simulink model "StateMachine_v3"  (R2015a)
settings: Solver=ode1  StartTime=0.0  StopTime=Inf  FixedStep=0.001  RelTol=1e-3
PostLoadFcn:
  | , if any(exist('dsrtsu_mdlpostloadfcn', 'file') == [2, 3, 6]), try dsrtsu_mdlpostloadfcn('Execute', bdroot); catch fprintf('Error in PostLoadFcn (dsrtsu_mdlpostloadfcn) for model "%s":\n %s\n', bdroot, lasterr); end, end,
libraries: rtican x25, rti1401lib_adc_type4 x16, rti1401lib_dio_type3 x16, rtilib1401 x1
(part 4 of 6)

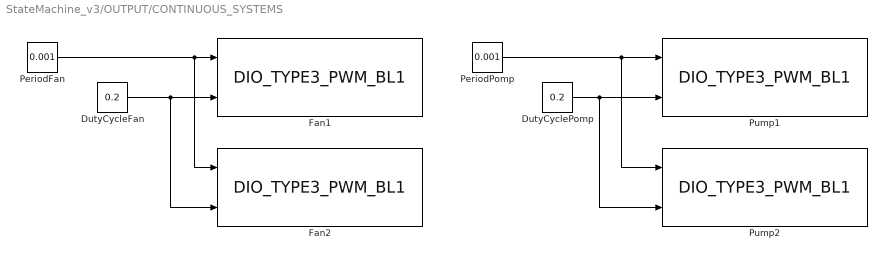
== system StateMachine_v3/OUTPUT/CONTINUOUS_SYSTEMS ==
  DutyCycleFan : Constant  Value=0.2
  DutyCyclePomp : Constant  Value=0.2
  Fan1 : rti1401lib_dio_type3/DIO_TYPE3_PWM_BL1  DSProperties=struct('RTI',struct('Version',uint32(2),'BlockType',struct('isSLSource',uint8(0),'isSLSink',uint8(1),'isHWSource',uint8(0),'isHWSink',uint8(1),'isSetup',uint8(0),'isInline',uint8(1),'isNonInline',uint8(0),'isInterrupt',uint8(0),'isChannelwise',uint8(1)),'IOBoardType',{{'DS1401','STD','DIOT3'}},'UnitType','PWM','Identifier','PWM','DialogType','ML','BlockSet','NONE','SlaveProcessor','NONE'))  RTIBlockInterface=struct('InputPortsWidth',int32([1 1]),'InputPortsActive',[1 1],'InputPortsName',{{'Period',['Duty Cycle']}},'BlockDisplay',{{['DIO TP3 PWM\nModule: 1\nPort: 1\nChannel: 3'],'center'}},'IconTransparency','on','InitLevel',3,'DialogFcn','rti1401stddiot3pwmgui','BlockName',struct('Token',{{'DIO_TYPE3_PWM_BL1'}}))  RTIBlockParameters=struct('ModuleNo',{{1,'OFF',[1 16]}},'PortNo',{{1,'OFF',[1 3]}},'ChannelNo',{{3,'OFF',[1 16]}},'SupplyRailsCh',{{[1 1],'OFF',[0 1 0 1]}},'UpdateMode',{{1,'ON',[1 2]}},'PeriodRange',{{7,'OFF',[1 16]}},'DutyCycleInit',{{'0','OFF',[0 1]}},'PeriodInit',{{'5e-05','OFF',[]}},'TerminationMode',{{0,'OFF',[0 1]}},'OutputTermValidate',{{0,'OFF',[0 1]}},'OutputTermBuildCheck',{{0,'OFF',[]}},'DutyCycleTerm',{{'0','OFF',[0 1]}},'PeriodTerm',{{'5e-05','OFF',[]}},'TLCFileName',{{'rti1401dio_t3_pwm','OFF',[]}},'EnableInterrupt',{{0,'OFF',[0 1]}},'TriggerEdgeType',{{1,'OFF',[1 3]}})  RTISFcnParameters=struct('ModuleNo','int32','PortNo','int16','ChannelNo','int16','SupplyRailsCh','int16','UpdateMode','int16','PeriodRange','int16','DutyCycleInit','double','PeriodInit','double','TerminationMode','int16','OutputTermValidate','int16','DutyCycleTerm','double','PeriodTerm','double','TLCFileName','char','EnableInterrupt','int16','TriggerEdgeType','int32')  RTIBlockParaDefault=struct('ModuleNo',1,'PortNo',1,'ChannelNo',1,'SupplyRailsCh',[1 1],'UpdateMode',1,'PeriodRange',7,'DutyCycleInit',0,'PeriodInit',5e-05,'TerminationMode',0,'OutputTermValidate',0,'OutputTermBuildCheck',0,'DutyCycleTerm',0,'PeriodTerm',5e-05,'TLCFileName','rti1401dio_t3_pwm','EnableInterrupt',0,'TriggerEdgeType',1)
  Fan2 : rti1401lib_dio_type3/DIO_TYPE3_PWM_BL1  DSProperties=struct('RTI',struct('Version',uint32(2),'BlockType',struct('isSLSource',uint8(0),'isSLSink',uint8(1),'isHWSource',uint8(0),'isHWSink',uint8(1),'isSetup',uint8(0),'isInline',uint8(1),'isNonInline',uint8(0),'isInterrupt',uint8(0),'isChannelwise',uint8(1)),'IOBoardType',{{'DS1401','STD','DIOT3'}},'UnitType','PWM','Identifier','PWM','DialogType','ML','BlockSet','NONE','SlaveProcessor','NONE'))  RTIBlockInterface=struct('InputPortsWidth',int32([1 1]),'InputPortsActive',[1 1],'InputPortsName',{{'Period',['Duty Cycle']}},'BlockDisplay',{{['DIO TP3 PWM\nModule: 1\nPort: 1\nChannel: 4'],'center'}},'IconTransparency','on','InitLevel',3,'DialogFcn','rti1401stddiot3pwmgui','BlockName',struct('Token',{{'DIO_TYPE3_PWM_BL1'}}))  RTIBlockParameters=struct('ModuleNo',{{1,'OFF',[1 16]}},'PortNo',{{1,'OFF',[1 3]}},'ChannelNo',{{4,'OFF',[1 16]}},'SupplyRailsCh',{{[1 1],'OFF',[0 1 0 1]}},'UpdateMode',{{1,'ON',[1 2]}},'PeriodRange',{{7,'OFF',[1 16]}},'DutyCycleInit',{{'0','OFF',[0 1]}},'PeriodInit',{{'5e-05','OFF',[]}},'TerminationMode',{{0,'OFF',[0 1]}},'OutputTermValidate',{{0,'OFF',[0 1]}},'OutputTermBuildCheck',{{0,'OFF',[]}},'DutyCycleTerm',{{'0','OFF',[0 1]}},'PeriodTerm',{{'5e-05','OFF',[]}},'TLCFileName',{{'rti1401dio_t3_pwm','OFF',[]}},'EnableInterrupt',{{0,'OFF',[0 1]}},'TriggerEdgeType',{{1,'OFF',[1 3]}})  RTISFcnParameters=struct('ModuleNo','int32','PortNo','int16','ChannelNo','int16','SupplyRailsCh','int16','UpdateMode','int16','PeriodRange','int16','DutyCycleInit','double','PeriodInit','double','TerminationMode','int16','OutputTermValidate','int16','DutyCycleTerm','double','PeriodTerm','double','TLCFileName','char','EnableInterrupt','int16','TriggerEdgeType','int32')  RTIBlockParaDefault=struct('ModuleNo',1,'PortNo',1,'ChannelNo',1,'SupplyRailsCh',[1 1],'UpdateMode',1,'PeriodRange',7,'DutyCycleInit',0,'PeriodInit',5e-05,'TerminationMode',0,'OutputTermValidate',0,'OutputTermBuildCheck',0,'DutyCycleTerm',0,'PeriodTerm',5e-05,'TLCFileName','rti1401dio_t3_pwm','EnableInterrupt',0,'TriggerEdgeType',1)
  PeriodFan : Constant  Value=0.001
  PeriodPomp : Constant  Value=0.001
  Pump1 : rti1401lib_dio_type3/DIO_TYPE3_PWM_BL1  DSProperties=struct('RTI',struct('Version',uint32(2),'BlockType',struct('isSLSource',uint8(0),'isSLSink',uint8(1),'isHWSource',uint8(0),'isHWSink',uint8(1),'isSetup',uint8(0),'isInline',uint8(1),'isNonInline',uint8(0),'isInterrupt',uint8(0),'isChannelwise',uint8(1)),'IOBoardType',{{'DS1401','STD','DIOT3'}},'UnitType','PWM','Identifier','PWM','DialogType','ML','BlockSet','NONE','SlaveProcessor','NONE'))  RTIBlockInterface=struct('InputPortsWidth',int32([1 1]),'InputPortsActive',[1 1],'InputPortsName',{{'Period',['Duty Cycle']}},'BlockDisplay',{{['DIO TP3 PWM\nModule: 1\nPort: 1\nChannel: 5'],'center'}},'IconTransparency','on','InitLevel',3,'DialogFcn','rti1401stddiot3pwmgui','BlockName',struct('Token',{{'DIO_TYPE3_PWM_BL1'}}))  RTIBlockParameters=struct('ModuleNo',{{1,'OFF',[1 16]}},'PortNo',{{1,'OFF',[1 3]}},'ChannelNo',{{5,'OFF',[1 16]}},'SupplyRailsCh',{{[1 1],'OFF',[0 1 0 1]}},'UpdateMode',{{1,'ON',[1 2]}},'PeriodRange',{{7,'OFF',[1 16]}},'DutyCycleInit',{{'0','OFF',[0 1]}},'PeriodInit',{{'5e-05','OFF',[]}},'TerminationMode',{{0,'OFF',[0 1]}},'OutputTermValidate',{{0,'OFF',[0 1]}},'OutputTermBuildCheck',{{0,'OFF',[]}},'DutyCycleTerm',{{'0','OFF',[0 1]}},'PeriodTerm',{{'5e-05','OFF',[]}},'TLCFileName',{{'rti1401dio_t3_pwm','OFF',[]}},'EnableInterrupt',{{0,'OFF',[0 1]}},'TriggerEdgeType',{{1,'OFF',[1 3]}})  RTISFcnParameters=struct('ModuleNo','int32','PortNo','int16','ChannelNo','int16','SupplyRailsCh','int16','UpdateMode','int16','PeriodRange','int16','DutyCycleInit','double','PeriodInit','double','TerminationMode','int16','OutputTermValidate','int16','DutyCycleTerm','double','PeriodTerm','double','TLCFileName','char','EnableInterrupt','int16','TriggerEdgeType','int32')  RTIBlockParaDefault=struct('ModuleNo',1,'PortNo',1,'ChannelNo',1,'SupplyRailsCh',[1 1],'UpdateMode',1,'PeriodRange',7,'DutyCycleInit',0,'PeriodInit',5e-05,'TerminationMode',0,'OutputTermValidate',0,'OutputTermBuildCheck',0,'DutyCycleTerm',0,'PeriodTerm',5e-05,'TLCFileName','rti1401dio_t3_pwm','EnableInterrupt',0,'TriggerEdgeType',1)
  Pump2 : rti1401lib_dio_type3/DIO_TYPE3_PWM_BL1  DSProperties=struct('RTI',struct('Version',uint32(2),'BlockType',struct('isSLSource',uint8(0),'isSLSink',uint8(1),'isHWSource',uint8(0),'isHWSink',uint8(1),'isSetup',uint8(0),'isInline',uint8(1),'isNonInline',uint8(0),'isInterrupt',uint8(0),'isChannelwise',uint8(1)),'IOBoardType',{{'DS1401','STD','DIOT3'}},'UnitType','PWM','Identifier','PWM','DialogType','ML','BlockSet','NONE','SlaveProcessor','NONE'))  RTIBlockInterface=struct('InputPortsWidth',int32([1 1]),'InputPortsActive',[1 1],'InputPortsName',{{'Period',['Duty Cycle']}},'BlockDisplay',{{['DIO TP3 PWM\nModule: 1\nPort: 1\nChannel: 6'],'center'}},'IconTransparency','on','InitLevel',3,'DialogFcn','rti1401stddiot3pwmgui','BlockName',struct('Token',{{'DIO_TYPE3_PWM_BL1'}}))  RTIBlockParameters=struct('ModuleNo',{{1,'OFF',[1 16]}},'PortNo',{{1,'OFF',[1 3]}},'ChannelNo',{{6,'OFF',[1 16]}},'SupplyRailsCh',{{[1 1],'OFF',[0 1 0 1]}},'UpdateMode',{{1,'ON',[1 2]}},'PeriodRange',{{7,'OFF',[1 16]}},'DutyCycleInit',{{'0','OFF',[0 1]}},'PeriodInit',{{'5e-05','OFF',[]}},'TerminationMode',{{0,'OFF',[0 1]}},'OutputTermValidate',{{0,'OFF',[0 1]}},'OutputTermBuildCheck',{{0,'OFF',[]}},'DutyCycleTerm',{{'0','OFF',[0 1]}},'PeriodTerm',{{'5e-05','OFF',[]}},'TLCFileName',{{'rti1401dio_t3_pwm','OFF',[]}},'EnableInterrupt',{{0,'OFF',[0 1]}},'TriggerEdgeType',{{1,'OFF',[1 3]}})  RTISFcnParameters=struct('ModuleNo','int32','PortNo','int16','ChannelNo','int16','SupplyRailsCh','int16','UpdateMode','int16','PeriodRange','int16','DutyCycleInit','double','PeriodInit','double','TerminationMode','int16','OutputTermValidate','int16','DutyCycleTerm','double','PeriodTerm','double','TLCFileName','char','EnableInterrupt','int16','TriggerEdgeType','int32')  RTIBlockParaDefault=struct('ModuleNo',1,'PortNo',1,'ChannelNo',1,'SupplyRailsCh',[1 1],'UpdateMode',1,'PeriodRange',7,'DutyCycleInit',0,'PeriodInit',5e-05,'TerminationMode',0,'OutputTermValidate',0,'OutputTermBuildCheck',0,'DutyCycleTerm',0,'PeriodTerm',5e-05,'TLCFileName','rti1401dio_t3_pwm','EnableInterrupt',0,'TriggerEdgeType',1)
  wires:
  DutyCycleFan/1 -> Fan2/2, Fan1/2
  PeriodFan/1 -> Fan2/1, Fan1/1
  DutyCyclePomp/1 -> Pump2/2, Pump1/2
  PeriodPomp/1 -> Pump2/1, Pump1/1

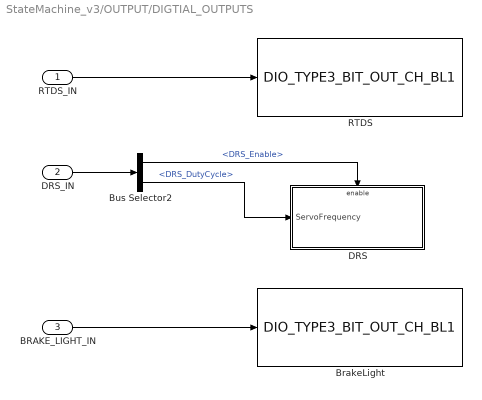
== system StateMachine_v3/OUTPUT/DIGTIAL_OUTPUTS ==
  RTDS_IN : Inport
  DRS_IN : Inport  Port=2
  BRAKE_LIGHT_IN : Inport  Port=3
  BrakeLight : rti1401lib_dio_type3/DIO_TYPE3_BIT_OUT_CH_BL1  DSProperties=struct('RTI',struct('Version',uint32(2),'BlockType',struct('isSLSource',uint8(0),'isSLSink',uint8(1),'isHWSource',uint8(0),'isHWSink',uint8(1),'isSetup',uint8(0),'isInline',uint8(1),'isNonInline',uint8(0),'isInterrupt',uint8(0),'isChannelwise',uint8(1)),'IOBoardType',{{'DS1401','STD','DIOT3'}},'UnitType','BIT','Identifier','BITOUTCH','DialogType','ML','BlockSet','NONE','SlaveProcessor','NONE'))  RTIBlockInterface=struct('InputPortsWidth',int32(1),'InputPortsActive',1,'InputPortsDataType',{{'SS_BOOLEAN'}},'InputPortsName',{{'In'}},'BlockDisplay',{{['DIO TP3 BIT OUT\n Channelwise\nModule: 1\nPort: 1\nChannel: 2'],'center'}},'IconTransparency','on','InitLevel',3,'DialogFcn','rti1401stddiot3bitoutchgui','BlockName',struct('Token',{{'DIO_TYPE3_BIT_OUT_CH_BL1'}}))  RTIBlockParameters=struct('ModuleNo',{{1,'OFF',[1 16]}},'PortNo',{{1,'OFF',[1 3]}},'ChannelNo',{{2,'OFF',[1 16]}},'OutputStateInit',{{0,'OFF',[0 1]}},'TerminationMode',{{0,'OFF',[0 1]}},'OutputStateTermValidate',{{0,'OFF',[0 1]}},'OutputStateTerm',{{0,'OFF',[0 1]}},'SupplyRailsCh',{{[1 1],'OFF',[0 1 0 1]}},'TLCFileName',{{'rti1401dio_t3_bit_out_ch','OFF',[]}},'EnableInterrupt',{{0,'OFF',[0 1]}},'TriggerEdgeType',{{1,'OFF',[1 3]}})  RTISFcnParameters=struct('ModuleNo','int32','PortNo','int16','ChannelNo','int16','SupplyRailsCh','int16','OutputStateInit','int16','TerminationMode','int16','OutputStateTermValidate','int16','OutputStateTerm','int16','TLCFileName','char','EnableInterrupt','int16','TriggerEdgeType','int32')  RTIBlockParaDefault=struct('ModuleNo',1,'PortNo',1,'ChannelNo',1,'OutputStateInit',0,'TerminationMode',0,'OutputStateTermValidate',0,'OutputStateTerm',0,'SupplyRailsCh',[1 1],'TLCFileName','rti1401dio_t3_bit_out_ch','EnableInterrupt',0,'TriggerEdgeType',1)
  Bus Selector2 : BusSelector  OutputSignals=DRS_Enable,DRS_DutyCycle
  DRS : Subsystem
  RTDS : rti1401lib_dio_type3/DIO_TYPE3_BIT_OUT_CH_BL1  DSProperties=struct('RTI',struct('Version',uint32(2),'BlockType',struct('isSLSource',uint8(0),'isSLSink',uint8(1),'isHWSource',uint8(0),'isHWSink',uint8(1),'isSetup',uint8(0),'isInline',uint8(1),'isNonInline',uint8(0),'isInterrupt',uint8(0),'isChannelwise',uint8(1)),'IOBoardType',{{'DS1401','STD','DIOT3'}},'UnitType','BIT','Identifier','BITOUTCH','DialogType','ML','BlockSet','NONE','SlaveProcessor','NONE'))  RTIBlockInterface=struct('InputPortsWidth',int32(1),'InputPortsActive',1,'InputPortsDataType',{{'SS_BOOLEAN'}},'InputPortsName',{{'In'}},'BlockDisplay',{{['DIO TP3 BIT OUT\n Channelwise\nModule: 1\nPort: 1\nChannel: 1'],'center'}},'IconTransparency','on','InitLevel',3,'DialogFcn','rti1401stddiot3bitoutchgui','BlockName',struct('Token',{{'DIO_TYPE3_BIT_OUT_CH_BL1'}}))  RTIBlockParameters=struct('ModuleNo',{{1,'OFF',[1 16]}},'PortNo',{{1,'OFF',[1 3]}},'ChannelNo',{{1,'OFF',[1 16]}},'OutputStateInit',{{0,'OFF',[0 1]}},'TerminationMode',{{0,'OFF',[0 1]}},'OutputStateTermValidate',{{0,'OFF',[0 1]}},'OutputStateTerm',{{0,'OFF',[0 1]}},'SupplyRailsCh',{{[1 1],'OFF',[0 1 0 1]}},'TLCFileName',{{'rti1401dio_t3_bit_out_ch','OFF',[]}},'EnableInterrupt',{{0,'OFF',[0 1]}},'TriggerEdgeType',{{1,'OFF',[1 3]}})  RTISFcnParameters=struct('ModuleNo','int32','PortNo','int16','ChannelNo','int16','SupplyRailsCh','int16','OutputStateInit','int16','TerminationMode','int16','OutputStateTermValidate','int16','OutputStateTerm','int16','TLCFileName','char','EnableInterrupt','int16','TriggerEdgeType','int32')  RTIBlockParaDefault=struct('ModuleNo',1,'PortNo',1,'ChannelNo',1,'OutputStateInit',0,'TerminationMode',0,'OutputStateTermValidate',0,'OutputStateTerm',0,'SupplyRailsCh',[1 1],'TLCFileName','rti1401dio_t3_bit_out_ch','EnableInterrupt',0,'TriggerEdgeType',1)
  wires:
  BRAKE_LIGHT_IN/1 -> BrakeLight/1
  DRS_IN/1 -> Bus Selector2/1
  RTDS_IN/1 -> RTDS/1
  Bus Selector2/1 -> DRS/Enable  "<DRS_Enable>"
  Bus Selector2/2 -> DRS/1(ServoFrequency)  "<DRS_DutyCycle>"
